simulink model "scheme_3A"  (R2021b)
settings: Solver=VariableStepAuto  StartTime=0.0  StopTime=100  RelTol=1e-3
model workspace (MAT data in the model file):
  Ti = 200
settings Model: Creator=valeria  LastModifiedBy=Ivan
settings SolverCC: AlgebraicLoopSolver=TrustRegion
settings DebuggingCC: SFMachineParentedDataDiag=warning

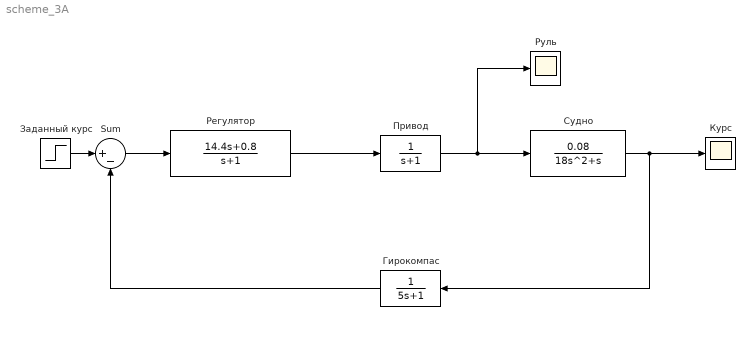
== system scheme_3A ==
  " Гирокомпас" : TransferFcn  Denominator=[5 1]
  Sum : Sum  Inputs=|+-
  Заданный курс : Step  Time=0  After=10  SampleTime=0
  Курс : Scope
  Привод : TransferFcn  Denominator=[1 1]
  Регулятор : TransferFcn  Numerator=[14.4 0.8]  Denominator=[1 1]
  Руль : Scope
  Судно : TransferFcn  Numerator=[0.08]  Denominator=[18 1 0]
  wires:
  Заданный курс/1 -> Sum/1
  Sum/1 -> Регулятор/1
  Судно/1 -> Курс/1, " Гирокомпас"/1
  " Гирокомпас"/1 -> Sum/2
  Привод/1 -> Руль/1, Судно/1
  Регулятор/1 -> Привод/1
